simulink model "TotemPole"  (R2022a)
settings: Solver=ode4  StartTime=0.0  StopTime=0.5  FixedStep=1e-7  RelTol=1e-3
undefined symbols (not defined in the file): C_totem, fs_PFC, Gcinf, Gcvinf, H, kx, L_totem, Rsense, Vm, wL, wLvv
libraries: spsSeriesRLCBranchLib x6, spsDiodeLib x4, spsMosfetLib x4, spsVoltageMeasurementLib x3, spsACVoltageSourceLib x1, hdlsllib x1, spsCurrentMeasurementLib x1, spsDCVoltageSourceLib x1, spsRMSLib x1, simulink x1, spspowerguiLib x1
settings Model: Creator=Aditya Bhalotia  LastModifiedBy=Aditya Bhalotia
settings DataIOCC: InspectSignalLogs=on  ReturnWorkspaceOutputs=off  LoggingToFile=on

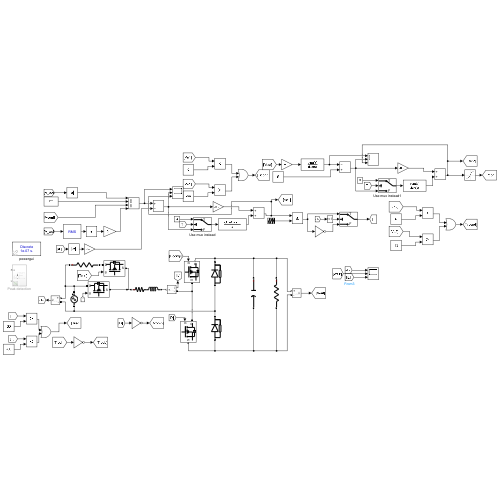
[thumbnail: Simulink's stored preview of the top-level diagram]
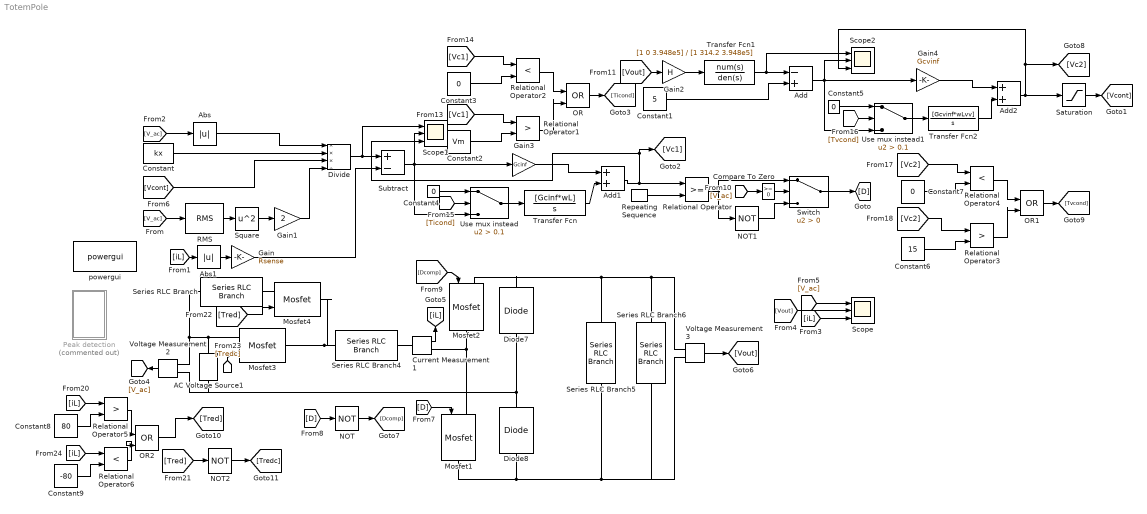
== system TotemPole ==
  AC Voltage Source1 : spsACVoltageSourceLib/AC Voltage Source  Amplitude=85*sqrt(2)  Phase=0  Frequency=50  SampleTime=0  Measurements=None  BusType=swing  Pref=10e3  Qref=0  Qmin=-inf  Qmax=+inf
  Abs : Abs  SaturateOnIntegerOverflow=off
  Abs1 : Abs  SaturateOnIntegerOverflow=off
  Add : Sum  Inputs=-+
  Add1 : Sum
  Add2 : Sum
  Compare To Zero : hdlsllib/Logic and Bit Operations/Compare To Zero  relop=>=  OutDataTypeStr=boolean
      settings: SourceProductBaseCode=SL
  Constant : Constant  Value=kx
  Constant1 : Constant  Value=5
  Constant2 : Constant  Value=Vm
  Constant{3..5,7} (4 alike) : Constant  Value=0
  Constant6 : Constant  Value=15
  Constant8 : Constant  Value=80
  Constant9 : Constant  Value=-80
  Current Measurement1 : spsCurrentMeasurementLib/Current Measurement  PhasorSimulation=off  OutputType=Complex  PSBequivalent=0
  Diode7 : spsDiodeLib/Diode  Ron=0.001  Lon=0  Vf=0  IC=0  UseSnubber=0  Rs=50e3  Cs=inf  Measurements=off
  Diode8 : spsDiodeLib/Diode  Ron=0.001  Lon=0  Vf=0  IC=0  UseSnubber=0  Rs=50e3  Cs=inf  Measurements=off
  Divide : Product  Inputs=***/
  Gain : Gain  Gain=Rsense
  Gain1 : Gain  Gain=2
  Gain2 : Gain  Gain=H
  Gain3 : Gain  Gain=Gcinf
  Gain4 : Gain  Gain=Gcvinf
  Mosfet{1..4} (4 alike) : spsMosfetLib/Mosfet  Ron=0.0001  Lon=0  Rd=0.0001  Vfd=0  IC=0  Rs=50e4  Cs=inf  Measurements=off
  NOT : Logic  Operator=NOT  IconShape=distinctive  AllPortsSameDT=off  OutDataTypeStr=boolean
  NOT1 : Logic  Operator=NOT  IconShape=distinctive  AllPortsSameDT=off  OutDataTypeStr=boolean
  NOT2 : Logic  Operator=NOT  IconShape=distinctive  AllPortsSameDT=off  OutDataTypeStr=boolean
  OR : Logic  Operator=OR  IconShape=distinctive  AllPortsSameDT=off  OutDataTypeStr=boolean
  OR1 : Logic  Operator=OR  IconShape=distinctive  AllPortsSameDT=off  OutDataTypeStr=boolean
  OR2 : Logic  Operator=OR  IconShape=distinctive  AllPortsSameDT=off  OutDataTypeStr=boolean
  Peak detection : Subsystem  Commented=on
  RMS : spsRMSLib/RMS  TrueRMS=off  Freq=50  RMSInit=220  Ts=0
  Relational Operator : RelationalOperator  OutDataTypeStr=boolean  RndMeth=Simplest  InputSameDT=off
  Relational Operator1 : RelationalOperator  Operator=>  OutDataTypeStr=boolean  RndMeth=Simplest  InputSameDT=off
  Relational Operator2 : RelationalOperator  Operator=<  OutDataTypeStr=boolean  RndMeth=Simplest  InputSameDT=off
  Relational Operator3 : RelationalOperator  Operator=>  OutDataTypeStr=boolean  RndMeth=Simplest  InputSameDT=off
  Relational Operator4 : RelationalOperator  Operator=<  OutDataTypeStr=boolean  RndMeth=Simplest  InputSameDT=off
  Relational Operator5 : RelationalOperator  Operator=>  OutDataTypeStr=boolean  RndMeth=Simplest  InputSameDT=off
  Relational Operator6 : RelationalOperator  Operator=<  OutDataTypeStr=boolean  RndMeth=Simplest  InputSameDT=off
  Repeating Sequence : simulink/Sources/Repeating Sequence  rep_seq_t=[0 1/fs_PFC]  rep_seq_y=[0 Vm]
  Saturation : Saturate  UpperLimit=15  LowerLimit=0
  Scope : Scope  NumInputPorts=3
  Scope1 : Scope  NumInputPorts=3
  Scope2 : Scope  NumInputPorts=3
  Series RLC Branch : spsSeriesRLCBranchLib/Series RLC Branch  LConnTagsString=__new0  RConnTagsString=__new0  BranchType=R  Resistance=5  Inductance=1e-3  SetiL0=off  InitialCurrent=0  Capacitance=1e-6  Setx0=off  InitialVoltage=0  Measurements=None
  Series RLC Branch4 : spsSeriesRLCBranchLib/Series RLC Branch  LConnTagsString=__new0  RConnTagsString=__new0  BranchType=RL  Resistance=0.2  Inductance=L_totem  SetiL0=off  InitialCurrent=0  Capacitance=1e-6  Setx0=off  InitialVoltage=0  Measurements=None
  Series RLC Branch5 : spsSeriesRLCBranchLib/Series RLC Branch  LConnTagsString=__new0  RConnTagsString=__new0  BranchType=C  Resistance=1  Inductance=1e-3  SetiL0=off  InitialCurrent=0  Capacitance=C_totem  Setx0=off  InitialVoltage=0  Measurements=None
  Series RLC Branch6 : spsSeriesRLCBranchLib/Series RLC Branch  LConnTagsString=__new0  RConnTagsString=__new0  BranchType=R  Resistance=44.4444  Inductance=1e-3  SetiL0=off  InitialCurrent=0  Capacitance=1e-6  Setx0=off  InitialVoltage=0  Measurements=Branch voltage
  Square : Math  Operator=square  OutputSignalType=real
  Subtract : Sum  Inputs=+-
  Switch : Switch  Criteria=u2 > Threshold  SaturateOnIntegerOverflow=off  InputSameDT=off
  Transfer Fcn : TransferFcn  Numerator=[Gcinf*wL]  Denominator=[1 0]
  Transfer Fcn1 : TransferFcn  Numerator=[1 0 3.948e5]  Denominator=[1 314.2 3.948e5]
  Transfer Fcn2 : TransferFcn  Numerator=[Gcvinf*wLvv]  Denominator=[1 0]
  Use mux instead : Switch  Criteria=u2 > Threshold  Threshold=0.1  SaturateOnIntegerOverflow=off  InputSameDT=off
  Use mux instead1 : Switch  Criteria=u2 > Threshold  Threshold=0.1  SaturateOnIntegerOverflow=off  InputSameDT=off
  Voltage Measurement2 : spsVoltageMeasurementLib/Voltage Measurement  PhasorSimulation=off  OutputType=Complex  PSBequivalent=0
  Voltage Measurement3 : spsVoltageMeasurementLib/Voltage Measurement  PhasorSimulation=off  OutputType=Complex  PSBequivalent=0
  powergui : spspowerguiLib/powergui  Priority=1  SimulationMode=Discrete  SampleTime=1e-7  frequency=60  Iterations=50  frequencyindice=0  Pbase=100e6  ErrMax=1e-4  UnitsV=kV  UnitsW=MW  buscounter=0  FunctionMessages=off  echomessages=off  EnableUseOfTLC=off  CurrentSourceSwitches=off  DisableSnubberDevices=off  DisableRonSwitches=off  DisableVfSwitches=off  DisplayEquations=off  AutomaticDiscreteSolvers=off  SolverType=Tustin/Backward Euler (TBE)  Interpol=off  ExternalGateDelay=off  methode=off  Ts=100  x0status=blocks  SPID=on  SwTol=0  HookPort=off  NonlinearTolerance=1e-4  nMaxIteration=100  ContinueOnMaxIteration=off  RestoreLinks=warning  ResistiveCurrentMeasurement=off  Frange=[0:2:500]  Ylog=off  Xlog=on  ShowGrid=off  save=off  variable=ZData  structure=0  ZoomFFT=off  StartTime=0.0  cycles=1  DisplayStyle=1  fundamental=60  FreqAxis=off  MaxFrequency=1000  frequencyindicesteady=1  RmsSteady=1  display=off
  wires:
  Repeating Sequence/1 -> Relational Operator/2
  Relational Operator/1 -> NOT1/1, Switch/1
  [V_ac] -> Abs/1
  Constant/1 -> Divide/2
  [Vcont] -> Divide/3
  [iL] -> Abs1/1
  [Vout] -> Scope/2
  [V_ac] -> Scope/1
  [iL] -> Scope/3
  Current Measurement1/1 -> [iL]
  Voltage Measurement3/1 -> [Vout]
  [D] -> Mosfet1/1
  Voltage Measurement2/1 -> [V_ac]
  [D] -> NOT/1
  NOT/1 -> [Dcomp]
  [Dcomp] -> Mosfet2/1
  NOT1/1 -> Switch/3
  [V_ac] -> Compare To Zero/1
  Compare To Zero/1 -> Switch/2
  Switch/1 -> [D]
  Abs/1 -> Divide/1
  Abs1/1 -> Gain/1
  RMS/1 -> Square/1
  Square/1 -> Gain1/1
  Gain1/1 -> Divide/4
  [V_ac] -> RMS/1
  Saturation/1 -> [Vcont]
  Divide/1 -> Scope1/1, Subtract/1
  Gain/1 -> Subtract/2
  Subtract/1 -> Scope1/2, Gain3/1, Use mux instead/3
  Gain3/1 -> Add1/1
  Transfer Fcn/1 -> Add1/2
  Add1/1 -> Scope1/3, [Vc1], Relational Operator/1
  [Vc1] -> Relational Operator1/1
  Constant2/1 -> Relational Operator1/2
  Constant3/1 -> Relational Operator2/2
  [Vc1] -> Relational Operator2/1
  Relational Operator2/1 -> OR/1
  Relational Operator1/1 -> OR/2
  Use mux instead/1 -> Transfer Fcn/1
  OR/1 -> [Ticond]
  [Ticond] -> Use mux instead/2
  Constant4/1 -> Use mux instead/1
  [Vout] -> Gain2/1
  Constant1/1 -> Add/2
  Gain2/1 -> Transfer Fcn1/1
  [Tvcond] -> Use mux instead1/2
  Gain4/1 -> Add2/1
  Transfer Fcn2/1 -> Add2/2
  Use mux instead1/1 -> Transfer Fcn2/1
  Constant5/1 -> Use mux instead1/1
  Constant7/1 -> Relational Operator4/2
  [Vc2] -> Relational Operator4/1
  Relational Operator3/1 -> OR1/2
  Relational Operator4/1 -> OR1/1
  OR1/1 -> [Tvcond]
  Constant6/1 -> Relational Operator3/2
  [Vc2] -> Relational Operator3/1
  Add2/1 -> Saturation/1, Scope2/3, [Vc2]
  [iL] -> Relational Operator5/1
  Constant8/1 -> Relational Operator5/2
  [Tred] -> NOT2/1
  NOT2/1 -> [Tredc]
  [Tred] -> Mosfet4/1
  [Tredc] -> Mosfet3/1
  Constant9/1 -> Relational Operator6/2
  [iL] -> Relational Operator6/1
  Relational Operator5/1 -> OR2/1
  Relational Operator6/1 -> OR2/2
  OR2/1 -> [Tred]
  Transfer Fcn1/1 -> Scope2/1, Add/1
  Add/1 -> Scope2/2, Use mux instead1/3, Gain4/1
  connections:
  Diode8/RConn1 -- AC Voltage Source1/LConn1 -- Voltage Measurement2/LConn2 -- Diode7/LConn1
  Series RLC Branch5/RConn1 -- Series RLC Branch6/RConn1 -- Voltage Measurement3/LConn2 -- Mosfet1/RConn1 -- Diode8/LConn1
  Series RLC Branch5/LConn1 -- Mosfet2/LConn1 -- Diode7/RConn1 -- Series RLC Branch6/LConn1 -- Voltage Measurement3/LConn1
  Current Measurement1/RConn1 -- Mosfet2/RConn1 -- Mosfet1/LConn1
  Voltage Measurement2/LConn1 -- Series RLC Branch/LConn1 -- AC Voltage Source1/RConn1 -- Mosfet3/LConn1
  Series RLC Branch4/RConn1 -- Current Measurement1/LConn1
  Mosfet3/RConn1 -- Mosfet4/RConn1 -- Series RLC Branch4/LConn1
  Series RLC Branch/RConn1 -- Mosfet4/LConn1

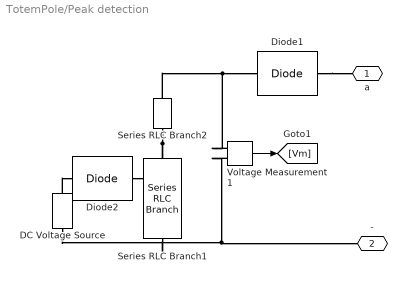
== system TotemPole/Peak detection ==
  DC Voltage Source : spsDCVoltageSourceLib/DC Voltage Source  Amplitude=1  Measurements=None
  Diode1 : spsDiodeLib/Diode  Ron=0.001  Lon=0  Vf=0  IC=0  UseSnubber=0  Rs=inf  Cs=inf  Measurements=off
  Diode2 : spsDiodeLib/Diode  Ron=0.001  Lon=0  Vf=0  IC=0  UseSnubber=0  Rs=inf  Cs=inf  Measurements=off
  Series RLC Branch1 : spsSeriesRLCBranchLib/Series RLC Branch  LConnTagsString=__new0  RConnTagsString=__new0  BranchType=C  Resistance=1  Inductance=1e-3  SetiL0=off  InitialCurrent=0  Capacitance=100e-6  Setx0=on  InitialVoltage=0  Measurements=None
  Series RLC Branch2 : spsSeriesRLCBranchLib/Series RLC Branch  LConnTagsString=__new0  RConnTagsString=__new0  BranchType=R  Resistance=2e-3  Inductance=1e-3  SetiL0=off  InitialCurrent=0  Capacitance=1e-6  Setx0=off  InitialVoltage=0  Measurements=Branch voltage
  Voltage Measurement1 : spsVoltageMeasurementLib/Voltage Measurement  PhasorSimulation=off  OutputType=Complex  PSBequivalent=0
  a : PMIOPort  Side=Left
  - : PMIOPort  Port=2  Side=Left
  wires:
  Voltage Measurement1/1 -> [Vm]
  connections:
  Voltage Measurement1/LConn2 -- DC Voltage Source/LConn1 -- Series RLC Branch1/RConn1 -- -/RConn1
  Diode1/LConn1 -- a/RConn1
  Series RLC Branch2/LConn1 -- Voltage Measurement1/LConn1 -- Diode1/RConn1
  DC Voltage Source/RConn1 -- Diode2/LConn1
  Series RLC Branch2/RConn1 -- Diode2/RConn1 -- Series RLC Branch1/LConn1
